simulink model "lecture18_simulink"  (R2017a)
settings: Solver=VariableStepAuto  StartTime=0.0  StopTime=end_time  RelTol=1e-3
values from neighbouring files (symbols this model uses):
  psi_init = 0.1    [lecture18_matlab.m]
  T_MPC = 0.1    [lecture18_MPC_sfunction.m]    (also in lecture18_matlab.m)
  v0 = 25    [lecture16_matlab.m]    (also in lecture18_matlab.m = 1)
  x_init = 0    [lecture18_matlab.m]
  x_target = 1    [lecture18_matlab.m]
  y_init = 0    [lecture18_matlab.m]
  y_target = 0    [lecture18_matlab.m]
settings Model: Creator=COE User  LastModifiedBy=COE User

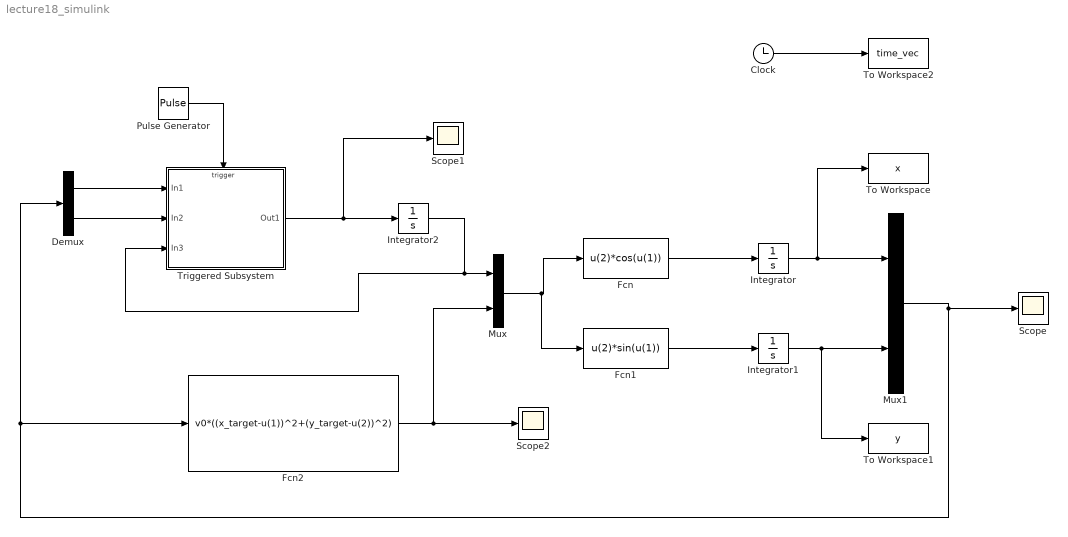
== system lecture18_simulink ==
  Clock : Clock
  Demux : Demux  Outputs=2
  Fcn : Fcn  Expr=u(2)*cos(u(1))
  Fcn1 : Fcn  Expr=u(2)*sin(u(1))
  Fcn2 : Fcn  Expr=v0*((x_target-u(1))^2+(y_target-u(2))^2)
  Integrator : Integrator  InitialCondition=x_init
  Integrator1 : Integrator  InitialCondition=y_init
  Integrator2 : Integrator  InitialCondition=psi_init
  Mux : Mux  Inputs=2
  Mux1 : Mux  Inputs=2
  Pulse Generator : DiscretePulseGenerator  PulseType=Time based  Period=T_MPC  PulseWidth=50
  Scope : Scope
  Scope1 : Scope
  Scope2 : Scope
  To Workspace : ToWorkspace  VariableName=x  SampleTime=-1
  To Workspace1 : ToWorkspace  VariableName=y  SampleTime=-1
  To Workspace2 : ToWorkspace  VariableName=time_vec  SampleTime=-1
  Triggered Subsystem : Subsystem  TreatAsAtomicUnit=on
  wires:
  Fcn/1 -> Integrator/1
  Fcn2/1 -> Mux/2, Scope2/1
  Triggered Subsystem/1(Out1) -> Scope1/1, Integrator2/1
  Integrator/1 -> To Workspace/1, Mux1/1
  Mux1/1 -> Scope/1, Demux/1, Fcn2/1
  Pulse Generator/1 -> Triggered Subsystem/Trigger
  Demux/1 -> Triggered Subsystem/1(In1)
  Demux/2 -> Triggered Subsystem/2(In2)
  Integrator2/1 -> Triggered Subsystem/3(In3), Mux/1
  Mux/1 -> Fcn1/1, Fcn/1
  Integrator1/1 -> To Workspace1/1, Mux1/2
  Fcn1/1 -> Integrator1/1
  Clock/1 -> To Workspace2/1

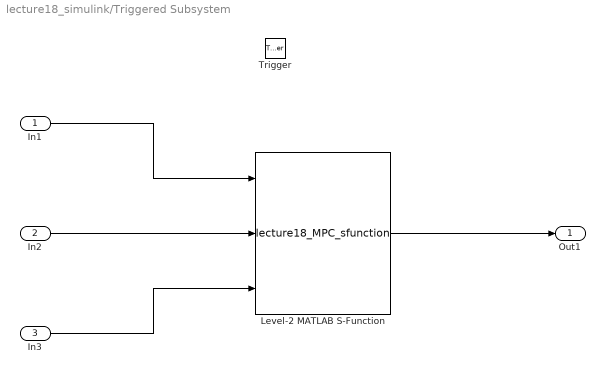
== system lecture18_simulink/Triggered Subsystem ==
  In1 : Inport
  In2 : Inport  Port=2
  In3 : Inport  Port=3
  Trigger : TriggerPort  VariantControl=Variant
  Level-2 MATLAB S-Function : M-S-Function  FunctionName=lecture18_MPC_sfunction
  Out1 : Outport
  wires:
  In1/1 -> Level-2 MATLAB S-Function/1
  In2/1 -> Level-2 MATLAB S-Function/2
  In3/1 -> Level-2 MATLAB S-Function/3
  Level-2 MATLAB S-Function/1 -> Out1/1
